simulink model "mdl_MoCo_Brake"  (R2019b)
settings: Solver=ode1  StartTime=0.0  StopTime=10.0  FixedStep=0.001  RelTol=1e-3
PostLoadFcn:
  | try
  | run([fileparts(which(gcs)) '\MoCo_Brake_Parameter'])
  | catch
  | end
undefined symbols (not defined in the file): accel_to_trq, brake_pres_exist_threshold, Brk_SSM_Decel_Lim, Brk_SSM_Hold_Grd_Lim, Brk_SSM_Release_Grd_Lim, D_brk, delay_brake_inc, delay_brake_inc_init, K_brk, K_brk_accel_dec, K_brk_trq_dec, T_brk_accel_dec, T_brk_trq_dec, w0_brk, w0_brkinit
settings Model: Creator=uid33443  LastModifiedBy=uid33443
settings RTWCC: Description=CarMaker Plug-in Model Target  SystemTargetFile=CarMaker.tlc  TemplateMakefile=CarMaker_unix-win64.tmf
settings CodeAppCC: MaxIdLength=127
settings STFCustomTargetCC: TargetLangStandard=C99 (ISO)  CombineOutputUpdateFcns=on  MatFileLogging=on  MultiInstanceERTCode=on  CodeInterfacePackaging=Reusable function  GenerateAllocFcn=on  SystemTargetFile=CarMaker.tlc
settings GRTTargetCC: ParMdlRefBuildCompliant=off  CompOptLevelCompliant=off  ConcurrentExecutionCompliant=off  MultiInstanceERTCode=on  CodeInterfacePackaging=Reusable function  CPPClassGenCompliant=off  GenerateAllocFcn=on  UseToolchainInfoCompliant=off  RTWCAPISignals=on  RTWCAPIParams=on  RTWCAPIStates=on

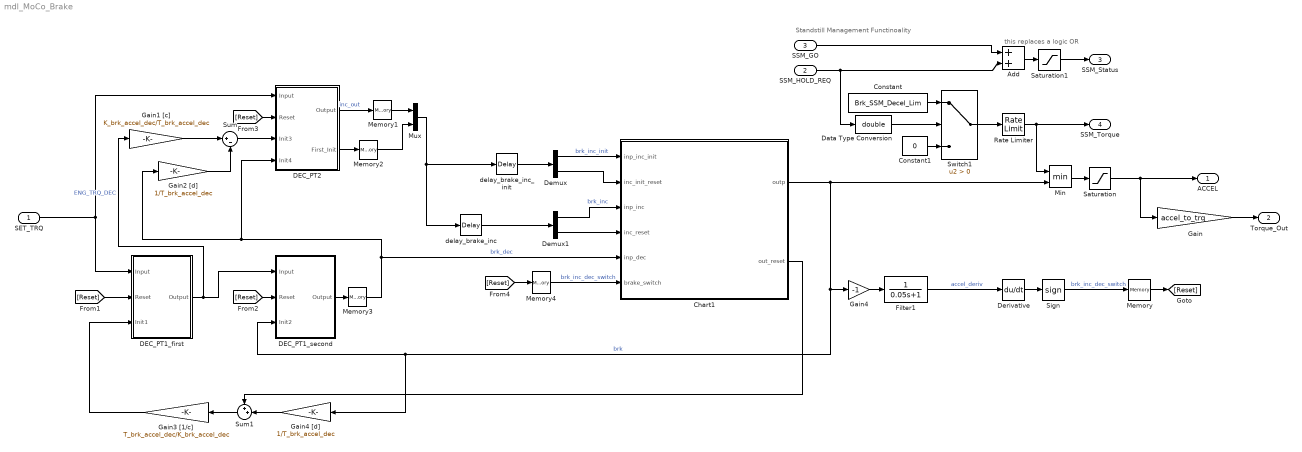
== system mdl_MoCo_Brake ==
  note: Standstill Management Functinoality
  note: this replaces a logic OR
  SET_TRQ : Inport
  SSM_HOLD_REQ : Inport  Port=2
  SSM_GO : Inport  Port=3
  Add : Sum
  Chart1 : Stateflow chart  TreatAsAtomicUnit=on
  Constant : Constant  Value=Brk_SSM_Decel_Lim
  Constant1 : Constant  Value=0
  DEC_PT1_first : Subsystem
  DEC_PT1_second : Subsystem
  DEC_PT2 : Subsystem
  Data Type Conversion : DataTypeConversion  OutDataTypeStr=double
  Demux : Demux  Outputs=2
  Demux1 : Demux  Outputs=2
  Derivative : Derivative
  Filter1 : TransferFcn  Denominator=[0.05 1]
  Gain : Gain  Gain=accel_to_trq
  Gain1 [c] : Gain  Gain=K_brk_accel_dec/T_brk_accel_dec
  Gain2 [d] : Gain  Gain=1/T_brk_accel_dec
  Gain3 [1/c] : Gain  Gain=T_brk_accel_dec/K_brk_accel_dec
  Gain4 : Gain  Gain=-1
  Gain4 [d] : Gain  Gain=1/T_brk_accel_dec
  Memory{,1..4} (5 alike) : Memory
  Min : MinMax  Inputs=2
  Mux : Mux  Inputs=2
  Rate Limiter : RateLimiter  RisingSlewLimit=Brk_SSM_Release_Grd_Lim  FallingSlewLimit=Brk_SSM_Hold_Grd_Lim  SampleTimeMode=inherited
  Saturation : Saturate  UpperLimit=0  LowerLimit=-inf
  Saturation1 : Saturate  UpperLimit=1  LowerLimit=0
  Sign : Signum
  Sum : Sum  Inputs=|+-
  Sum1 : Sum  Inputs=++|
  Switch1 : Switch  Criteria=u2 > Threshold
  delay_brake_inc : TransportDelay  DelayTime=delay_brake_inc  BufferSize=2048
  delay_brake_inc_init : TransportDelay  DelayTime=delay_brake_inc_init  BufferSize=2048
  ACCEL : Outport  VectorParamsAs1DForOutWhenUnconnected=off
  Torque_Out : Outport  Port=2  VectorParamsAs1DForOutWhenUnconnected=off
  SSM_Status : Outport  Port=3  VectorParamsAs1DForOutWhenUnconnected=off
  "SSM_Torque " : Outport  Port=4  VectorParamsAs1DForOutWhenUnconnected=off
  wires:
  Data Type Conversion/1 -> Switch1/2
  Saturation1/1 -> SSM_Status/1
  Demux/2 -> Chart1/2(inc_init_reset)
  Switch1/1 -> Rate Limiter/1
  Sum1/1 -> Gain3 [1/c]/1
  [Reset] -> DEC_PT1_first/2(Reset)
  Add/1 -> Saturation1/1
  Gain4/1 -> Filter1/1
  Gain2 [d]/1 -> Sum/2
  SSM_HOLD_REQ/1 -> Add/2, Data Type Conversion/1
  Memory2/1 -> Mux/2
  Constant/1 -> Switch1/1
  Gain/1 -> Torque_Out/1
  Rate Limiter/1 -> "SSM_Torque "/1, Min/1
  Sum/1 -> DEC_PT2/3(Init3)
  Mux/1 -> delay_brake_inc_init/1, delay_brake_inc/1
  [Reset] -> DEC_PT1_second/2(Reset)
  Gain4 [d]/1 -> Sum1/2
  delay_brake_inc/1 -> Demux1/1
  DEC_PT2/1(Output) -> Memory1/1  "inc_out"
  Demux1/2 -> Chart1/4(inc_reset)
  Filter1/1 -> Derivative/1  "accel_deriv"
  Min/1 -> Saturation/1
  Chart1/2(out_reset) -> Sum1/1
  DEC_PT1_first/1(Output) -> Gain1 [c]/1, DEC_PT1_second/1(Input)  "ENG_TRQ_DEC"
  Memory1/1 -> Mux/1
  Gain3 [1/c]/1 -> DEC_PT1_first/3(Init1)
  Gain1 [c]/1 -> Sum/1
  Memory4/1 -> Chart1/6(brake_switch)  "brk_inc_dec_switch"
  DEC_PT2/2(First_Init) -> Memory2/1
  Demux1/1 -> Chart1/3(inp_inc)  "brk_inc"
  Constant1/1 -> Switch1/3
  Demux/1 -> Chart1/1(inp_inc_init)  "brk_inc_init"
  Memory3/1 -> Chart1/5(inp_dec), Gain2 [d]/1, DEC_PT2/4(Init4)  "brk_dec"
  SET_TRQ/1 -> DEC_PT1_first/1(Input), DEC_PT2/1(Input)
  delay_brake_inc_init/1 -> Demux/1
  [Reset] -> DEC_PT2/2(Reset)
  DEC_PT1_second/1(Output) -> Memory3/1
  SSM_GO/1 -> Add/1
  Chart1/1(outp) -> Min/2, Gain4/1, DEC_PT1_second/3(Init2), Gain4 [d]/1  "brk"
  Saturation/1 -> ACCEL/1, Gain/1
  Derivative/1 -> Sign/1
  Memory/1 -> [Reset]
  Sign/1 -> Memory/1  "brk_inc_dec_switch"
  [Reset] -> Memory4/1

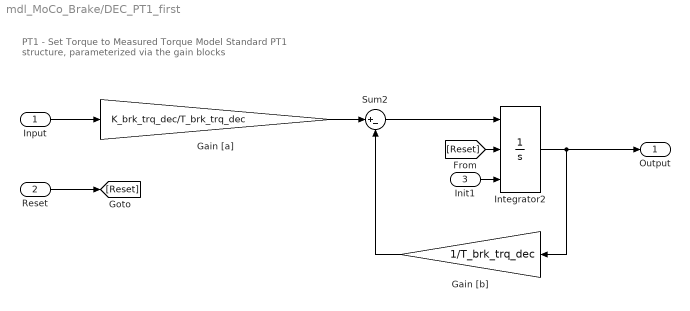
== system mdl_MoCo_Brake/DEC_PT1_first ==
  note: PT1 - Set Torque to Measured Torque Model
      | Standard PT1 structure, parameterized via the gain blocks
  Input : Inport
  Reset : Inport  Port=2
  Init1 : Inport  Port=3
  Gain [a] : Gain  Gain=K_brk_trq_dec/T_brk_trq_dec
  Gain [b] : Gain  Gain=1/T_brk_trq_dec
  Integrator2 : Integrator  ExternalReset=falling  InitialConditionSource=external
  Sum2 : Sum  Inputs=|+-
  Output : Outport  VectorParamsAs1DForOutWhenUnconnected=off
  wires:
  [Reset] -> Integrator2/2
  Init1/1 -> Integrator2/3
  Reset/1 -> [Reset]
  Gain [a]/1 -> Sum2/1
  Gain [b]/1 -> Sum2/2
  Input/1 -> Gain [a]/1
  Integrator2/1 -> Gain [b]/1, Output/1
  Sum2/1 -> Integrator2/1

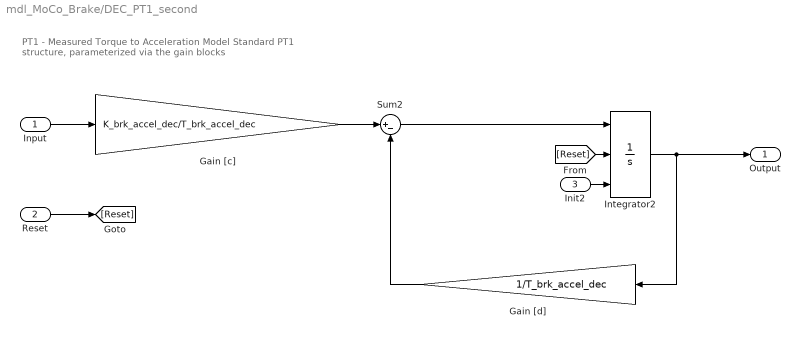
== system mdl_MoCo_Brake/DEC_PT1_second ==
  note: PT1 - Measured Torque to Acceleration Model
      | Standard PT1 structure, parameterized via the gain blocks
  Input : Inport
  Reset : Inport  Port=2
  Init2 : Inport  Port=3
  Gain [c] : Gain  Gain=K_brk_accel_dec/T_brk_accel_dec
  Gain [d] : Gain  Gain=1/T_brk_accel_dec
  Integrator2 : Integrator  ExternalReset=falling  InitialConditionSource=external
  Sum2 : Sum  Inputs=|+-
  Output : Outport  VectorParamsAs1DForOutWhenUnconnected=off
  wires:
  [Reset] -> Integrator2/2
  Init2/1 -> Integrator2/3
  Reset/1 -> [Reset]
  Gain [c]/1 -> Sum2/1
  Gain [d]/1 -> Sum2/2
  Input/1 -> Gain [c]/1
  Integrator2/1 -> Gain [d]/1, Output/1
  Sum2/1 -> Integrator2/1

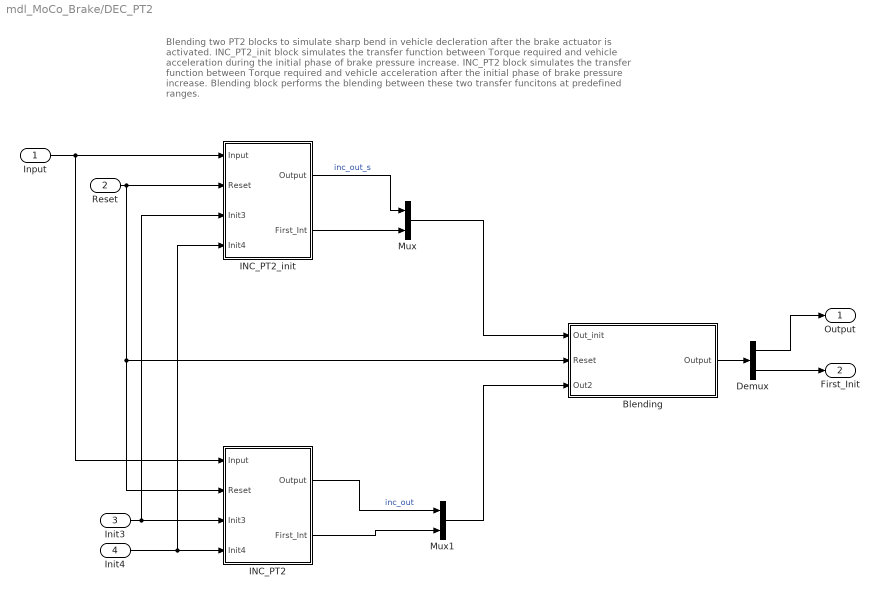
== system mdl_MoCo_Brake/DEC_PT2 ==
  note: Blending two PT2 blocks to simulate sharp bend in vehicle decleration after the brake actuator is activated.
      | INC_PT2_init block simulates the transfer function between Torque required and vehicle acceleration during the initial phase of brake pressure increase.
      | INC_PT2 block simulates the transfer function between Torque required and vehicle acceleration after the initial phase of brake pressure increase.
      | Blending block performs the blending between these two transfer funcitons at predefined ranges.
  Input : Inport
  Reset : Inport  Port=2
  Init3 : Inport  Port=3
  Init4 : Inport  Port=4
  Blending : Subsystem
  Demux : Demux  Outputs=2
  INC_PT2 : Subsystem
  INC_PT2_init : Subsystem
  Mux : Mux  Inputs=2
  Mux1 : Mux  Inputs=2
  Output : Outport  VectorParamsAs1DForOutWhenUnconnected=off
  First_Init : Outport  Port=2  VectorParamsAs1DForOutWhenUnconnected=off
  wires:
  Demux/2 -> First_Init/1
  Demux/1 -> Output/1
  Blending/1(Output) -> Demux/1
  Mux1/1 -> Blending/3(Out2)
  Mux/1 -> Blending/1(Out_init)
  INC_PT2_init/2(First_Int) -> Mux/2
  INC_PT2/1(Output) -> Mux1/1  "inc_out"
  INC_PT2_init/1(Output) -> Mux/1  "inc_out_s"
  Init4/1 -> INC_PT2/4(Init4), INC_PT2_init/4(Init4)
  Input/1 -> INC_PT2_init/1(Input), INC_PT2/1(Input)
  INC_PT2/2(First_Int) -> Mux1/2
  Reset/1 -> INC_PT2_init/2(Reset), Blending/2(Reset), INC_PT2/2(Reset)
  Init3/1 -> INC_PT2/3(Init3), INC_PT2_init/3(Init3)

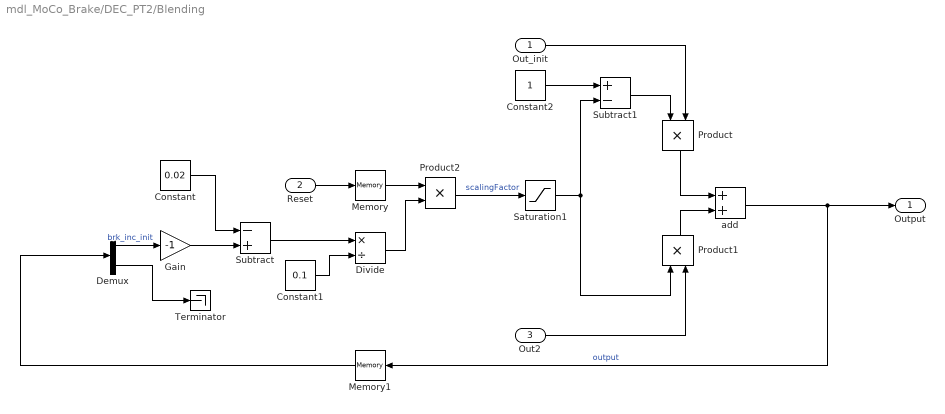
== system mdl_MoCo_Brake/DEC_PT2/Blending ==
  Out_init : Inport
  Reset : Inport  Port=2
  Out2 : Inport  Port=3
  Constant : Constant  Value=0.02
  Constant1 : Constant  Value=0.1
  Constant2 : Constant
  Demux : Demux  Outputs=2
  Divide : Product  Inputs=*/
  Gain : Gain  Gain=-1
  Memory : Memory
  Memory1 : Memory
  Product : Product
  Product1 : Product
  Product2 : Product
  Saturation1 : Saturate  UpperLimit=1  LowerLimit=0
  Subtract : Sum  Inputs=-+
  Subtract1 : Sum  Inputs=+-
  Terminator : Terminator
  add : Sum
  Output : Outport  VectorParamsAs1DForOutWhenUnconnected=off
  wires:
  add/1 -> Memory1/1, Output/1  "output"
  Product/1 -> add/1
  Gain/1 -> Subtract/2
  Constant1/1 -> Divide/2
  Saturation1/1 -> Subtract1/2, Product1/1
  Subtract/1 -> Divide/1
  Constant/1 -> Subtract/1
  Subtract1/1 -> Product/1
  Memory/1 -> Product2/1
  Product2/1 -> Saturation1/1  "scalingFactor"
  Product1/1 -> add/2
  Demux/2 -> Terminator/1
  Out_init/1 -> Product/2
  Reset/1 -> Memory/1
  Divide/1 -> Product2/2
  Constant2/1 -> Subtract1/1
  Demux/1 -> Gain/1  "brk_inc_init"
  Out2/1 -> Product1/2
  Memory1/1 -> Demux/1

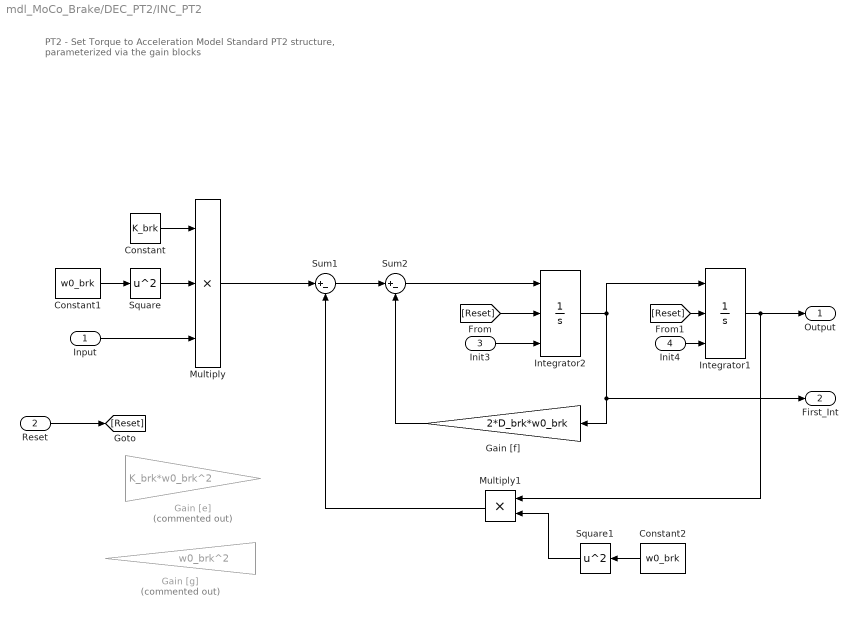
== system mdl_MoCo_Brake/DEC_PT2/INC_PT2 ==
  note: PT2 - Set Torque to Acceleration Model
      | Standard PT2 structure, parameterized via the gain blocks
  Input : Inport
  Reset : Inport  Port=2
  Init3 : Inport  Port=3
  Init4 : Inport  Port=4
  Constant : Constant  Value=K_brk
  Constant1 : Constant  Value=w0_brk
  Constant2 : Constant  Value=w0_brk
  Gain [e] : Gain  Commented=on  Gain=K_brk*w0_brk^2
  Gain [f] : Gain  Gain=2*D_brk*w0_brk
  Gain [g] : Gain  Commented=on  Gain=w0_brk^2
  Integrator1 : Integrator  ExternalReset=rising  InitialConditionSource=external
  Integrator2 : Integrator  ExternalReset=rising  InitialConditionSource=external
  Multiply : Product  Inputs=3
  Multiply1 : Product
  Square : Math  Operator=square  SaturateOnIntegerOverflow=on
  Square1 : Math  Operator=square  SaturateOnIntegerOverflow=on
  Sum1 : Sum  Inputs=|+-
  Sum2 : Sum  Inputs=|+-
  Output : Outport  VectorParamsAs1DForOutWhenUnconnected=off
  First_Int : Outport  Port=2  VectorParamsAs1DForOutWhenUnconnected=off
  wires:
  [Reset] -> Integrator1/2
  [Reset] -> Integrator2/2
  Init4/1 -> Integrator1/3
  Init3/1 -> Integrator2/3
  Reset/1 -> [Reset]
  Multiply1/1 -> Sum1/2
  Sum1/1 -> Sum2/1
  Integrator1/1 -> Multiply1/1, Output/1
  Gain [f]/1 -> Sum2/2
  Input/1 -> Multiply/3
  Integrator2/1 -> Gain [f]/1, First_Int/1, Integrator1/1
  Sum2/1 -> Integrator2/1
  Multiply/1 -> Sum1/1
  Constant1/1 -> Square/1
  Constant/1 -> Multiply/1
  Square/1 -> Multiply/2
  Constant2/1 -> Square1/1
  Square1/1 -> Multiply1/2

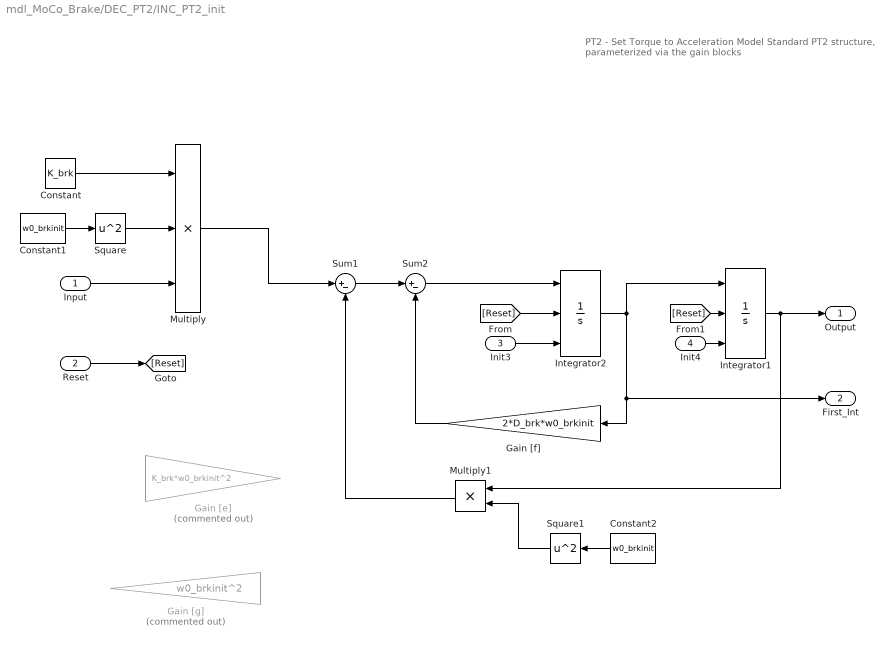
== system mdl_MoCo_Brake/DEC_PT2/INC_PT2_init ==
  note: PT2 - Set Torque to Acceleration Model
      | Standard PT2 structure, parameterized via the gain blocks
  Input : Inport
  Reset : Inport  Port=2
  Init3 : Inport  Port=3
  Init4 : Inport  Port=4
  Constant : Constant  Value=K_brk
  Constant1 : Constant  Value=w0_brkinit
  Constant2 : Constant  Value=w0_brkinit
  Gain [e] : Gain  Commented=on  Gain=K_brk*w0_brkinit^2
  Gain [f] : Gain  Gain=2*D_brk*w0_brkinit
  Gain [g] : Gain  Commented=on  Gain=w0_brkinit^2
  Integrator1 : Integrator  ExternalReset=rising  InitialConditionSource=external
  Integrator2 : Integrator  ExternalReset=rising  InitialConditionSource=external
  Multiply : Product  Inputs=3
  Multiply1 : Product
  Square : Math  Operator=square  SaturateOnIntegerOverflow=on
  Square1 : Math  Operator=square  SaturateOnIntegerOverflow=on
  Sum1 : Sum  Inputs=|+-
  Sum2 : Sum  Inputs=|+-
  Output : Outport  VectorParamsAs1DForOutWhenUnconnected=off
  First_Int : Outport  Port=2  VectorParamsAs1DForOutWhenUnconnected=off
  wires:
  Multiply/1 -> Sum1/1
  Sum2/1 -> Integrator2/1
  Integrator2/1 -> Integrator1/1, First_Int/1, Gain [f]/1
  Input/1 -> Multiply/3
  Gain [f]/1 -> Sum2/2
  Integrator1/1 -> Multiply1/1, Output/1
  Sum1/1 -> Sum2/1
  Multiply1/1 -> Sum1/2
  Reset/1 -> [Reset]
  Init3/1 -> Integrator2/3
  Init4/1 -> Integrator1/3
  [Reset] -> Integrator2/2
  [Reset] -> Integrator1/2
  Constant1/1 -> Square/1
  Square/1 -> Multiply/2
  Constant/1 -> Multiply/1
  Constant2/1 -> Square1/1
  Square1/1 -> Multiply1/2

== stateflow chart mdl_MoCo_Brake/Chart1 ==
  state dec
    entry: outp = inp_dec;
    during: outp = inp_dec;
  state Incresae phase with existing system pressure [group]
    state Inc_Trans
      entry: temp = inp_dec;
      during: outp = temp;
    state Inc_Trans1
      during: outp = inp_inc;
      out_reset = inc_reset;
    Inc_Trans -> Inc_Trans1 [order 1] : after(delay_brake_inc,sec)
  state Increase phase without existing system pressure [group]
    state Inc_Trans_init
      entry: temp = inp_dec;
      during: outp = temp;
    state Inc_init
      during: outp = inp_inc_init;
      out_reset = inc_init_reset;
    Inc_Trans_init -> Inc_init [order 1] : after(delay_brake_inc_init,sec)
  (default) -> dec
  dec -> Inc_Trans_init [order 1] : [(brake_switch == 1) & outp > (brake_pres_exist_threshold)]
  dec -> Inc_Trans [order 2] : [(brake_switch == 1) & outp <= (brake_pres_exist_threshold)]
  Inc_Trans_init -> dec [order 2] : [brake_switch == -1]
  Inc_init -> dec : [brake_switch == -1]
  Inc_Trans1 -> dec : [brake_switch == -1]
  Inc_Trans -> dec [order 2] : [brake_switch == -1]
  data: outp output; temp local; delay_brake_inc_init parameter; brake_pres_exist_threshold parameter; delay_brake_inc parameter; inp_inc_init input; inc_init_reset input; inp_inc input; inc_reset input; inp_dec input; brake_switch input; out_reset output
